simulink model "E5_Manual"  (R2019a)
settings: Solver=ode4  StartTime=0.0  StopTime=40  FixedStep=1e-3  RelTol=1e-2
libraries: simulink x2, simulink_extras x1
settings Model: Creator=anmay  LastModifiedBy=anmay
settings SolverCC: AlgebraicLoopSolver=LineSearch

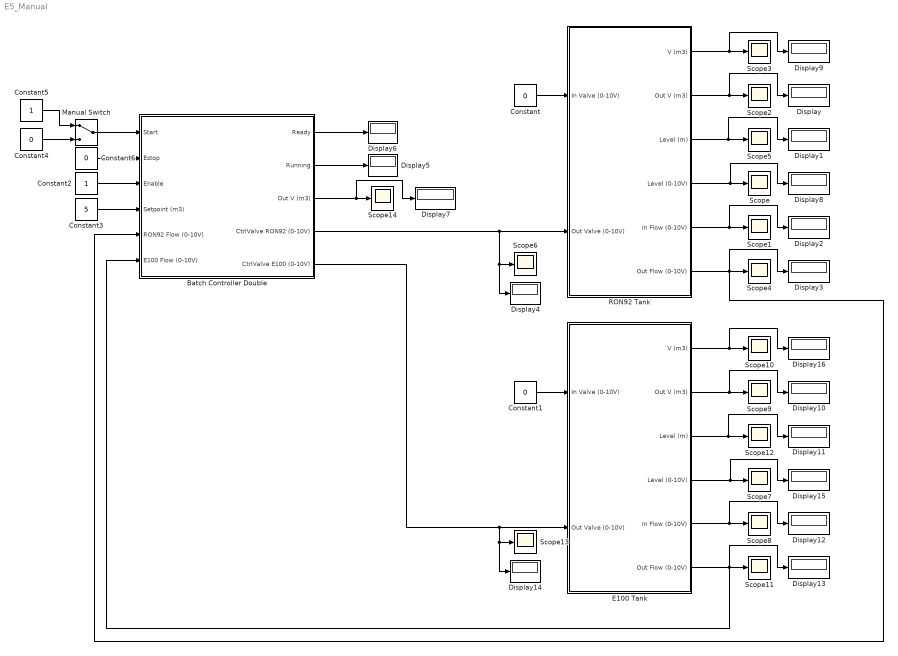
== system E5_Manual ==
  Batch Controller Double : Subsystem  mask{FlowMaxRON92=200, FlowMaxE100=100}
      mask prompts: FlowMaxRON92 "Lưu lượng tối đa RON92 (van mở 100%) (l/s)"; FlowMaxE100 "Lưu lượng tối đa E100 (van mở 100%) (l/s)"
  Constant{,1,4,6} (4 alike) : Constant  Value=0
  Constant2 : Constant
  Constant3 : Constant  Value=5
  Constant5 : Constant
  Display{,1..16} (17 alike) : Display
  E100 Tank : Subsystem  mask{InitialLevel=15, TankHeight=25, FlowMax=50, BaseArea=10, Tqt=0.1, EnableNoise=off, VarNoise=20}
      mask prompts: InitialLevel "Mức nhiên liệu ban đầu (m)"; TankHeight "Chiều cao của bể (m)"; FlowMax "Lưu lượng tối đa (van mở 100%) (l/s)"; BaseArea "Diện tích đáy (m2)"; Tqt "Hằng số quán tính của van (s)"; EnableNoise "Tạo nhiễu"; VarNoise "Phương sai của bộ tạo nhiễu"
  Manual Switch : ManualSwitch
  RON92 Tank : Subsystem  mask{InitialLevel=15, TankHeight=25, FlowMax=200, BaseArea=10, Tqt=0.2, EnableNoise=off, VarNoise=20}
      mask prompts: InitialLevel "Mức nhiên liệu ban đầu (m)"; TankHeight "Chiều cao của bể (m)"; FlowMax "Lưu lượng tối đa (van mở 100%) (l/s)"; BaseArea "Diện tích đáy (m2)"; Tqt "Hằng số quán tính của van (s)"; EnableNoise "Tạo nhiễu"; VarNoise "Phương sai của bộ tạo nhiễu"
  Scope{,1..14} (15 alike) : Scope
  wires:
  RON92 Tank/1(V (m3)) -> Display9/1, Scope3/1
  RON92 Tank/2(Out V (m3)) -> Scope2/1, Display/1
  RON92 Tank/3(Level (m)) -> Scope5/1, Display1/1
  RON92 Tank/6(Out Flow (0-10V)) -> Batch Controller Double/5(RON92 Flow (0-10V)), Display3/1, Scope4/1
  Batch Controller Double/4(CtrlValve RON92 (0-10V)) -> RON92 Tank/2(Out Valve (0-10V)), Display4/1, Scope6/1
  Batch Controller Double/2(Running) -> Display5/1
  RON92 Tank/4(Level (0-10V)) -> Scope/1, Display8/1
  Batch Controller Double/1(Ready) -> Display6/1
  RON92 Tank/5(In Flow (0-10V)) -> Display2/1, Scope1/1
  Constant/1 -> RON92 Tank/1(In Valve (0-10V))
  E100 Tank/5(In Flow (0-10V)) -> Display12/1, Scope8/1
  E100 Tank/3(Level (m)) -> Scope12/1, Display11/1
  E100 Tank/4(Level (0-10V)) -> Scope7/1, Display15/1
  Batch Controller Double/5(CtrlValve E100 (0-10V)) -> E100 Tank/2(Out Valve (0-10V)), Display14/1, Scope13/1
  E100 Tank/6(Out Flow (0-10V)) -> Batch Controller Double/6(E100 Flow (0-10V)), Display13/1, Scope11/1
  E100 Tank/1(V (m3)) -> Display16/1, Scope10/1
  Constant1/1 -> E100 Tank/1(In Valve (0-10V))
  E100 Tank/2(Out V (m3)) -> Scope9/1, Display10/1
  Constant4/1 -> Manual Switch/2
  Constant5/1 -> Manual Switch/1
  Constant2/1 -> Batch Controller Double/3(Enable)
  Constant6/1 -> Batch Controller Double/2(Estop)
  Constant3/1 -> Batch Controller Double/4(Setpoint (m3))
  Manual Switch/1 -> Batch Controller Double/1(Start)
  Batch Controller Double/3(Out V (m3)) -> Display7/1, Scope14/1

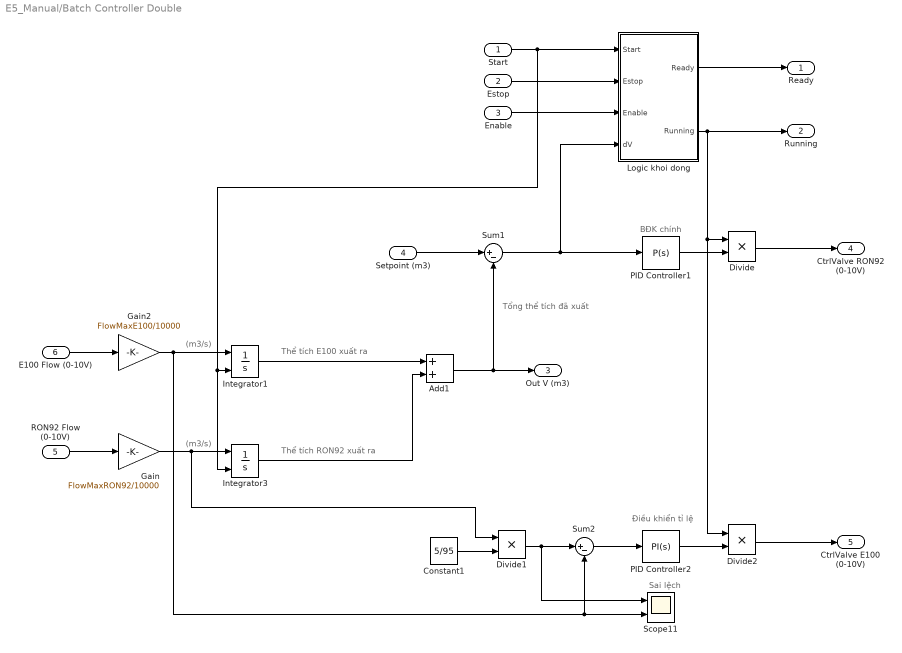
== system E5_Manual/Batch Controller Double ==
  note: (m3/s)
  note: BĐK chính
  note: Tổng thể tích đã xuất
  note: Điều khiển tỉ lệ
  note: Sai lệch
  note: Thể tích RON92 xuất ra
  note: Thể tích E100 xuất ra
  note: (m3/s)
  Start : Inport
  Estop : Inport  Port=2
  Enable : Inport  Port=3
  Setpoint (m3) : Inport  Port=4
  RON92 Flow (0-10V) : Inport  Port=5
  E100 Flow (0-10V) : Inport  Port=6
  Add1 : Sum
  Constant1 : Constant  Value=5/95
  Divide : Product  Inputs=**
  Divide1 : Product  Inputs=**
  Divide2 : Product  Inputs=**
  Gain : Gain  Gain=FlowMaxRON92/10000
  Gain2 : Gain  Gain=FlowMaxE100/10000
  Integrator1 : Integrator  ExternalReset=rising
  Integrator3 : Integrator  ExternalReset=rising
  Logic khoi dong : Subsystem
  PID Controller1 : simulink/Continuous/PID Controller  Controller=P  Form=Parallel  TimeDomain=Continuous-time  SampleTime=-1  IntegratorMethod=Forward Euler  FilterMethod=Forward Euler  ControllerParametersSource=internal  P=10  I=1  D=0  UseFilter=on  N=100  TunerSelectOption=Transfer Function Based (PID Tuner App)  InitialConditionSource=internal  InitialConditionForIntegrator=0  InitialConditionForFilter=0  DifferentiatorICPrevScaledInput=0  ExternalReset=none  TrackingMode=off  Kt=1  LimitOutput=on  UpperSaturationLimit=10  LowerSaturationLimit=0  LinearizeAsGain=on  AntiWindupMode=none  Kb=1  POutMin=[]  POutMax=[]  IOutMin=[]  IOutMax=[]  DOutMin=[]  DOutMax=[]  NOutMin=[]  NOutMax=[]  SumOutMin=[]  SumOutMax=[]  SaturationOutMin=[]  SaturationOutMax=[]  PParamMin=[]  PParamMax=[]  IParamMin=[]  IParamMax=[]  DParamMin=[]  DParamMax=[]  NParamMin=[]  NParamMax=[]  KbParamMin=[]  KbParamMax=[]  KtParamMin=[]  KtParamMax=[]  KbOutMin=[]  KbOutMax=[]  KtOutMin=[]  KtOutMax=[]  IntegratorOutMin=[]  IntegratorOutMax=[]  FilterOutMin=[]  FilterOutMax=[]  SumI1OutMin=[]  SumI1OutMax=[]  SumI2OutMin=[]  SumI2OutMax=[]  SumI3OutMin=[]  SumI3OutMax=[]  SumI4OutMin=[]  SumI4OutMax=[]  SumDOutMin=[]  SumDOutMax=[]  DifferentiatorOutMin=[]  DifferentiatorOutMax=[]  FilterDiffOutCoefMin=[]  FilterDiffOutCoefMax=[]  ReciprocalOutMin=[]  ReciprocalOutMax=[]  SumDenOutMin=[]  SumDenOutMax=[]  SumNumOutMin=[]  SumNumOutMax=[]  DivideOutMin=[]  DivideOutMax=[]  IntegratorContinuousStateAttributes=''  IntegratorStateMustResolveToSignalObject=off  IntegratorRTWStateStorageClass=Auto  FilterContinuousStateAttributes=''  FilterStateMustResolveToSignalObject=off  FilterRTWStateStorageClass=Auto  ParallelPVariant=InternalParameters  IdealPVariant=Disabled  IVariant=Disabled  DVariant=Disabled  IntegratorVariant=Disabled  SatVariant=Enabled  AWVariant=Disabled  PCopyVariant=Disabled  TRVariant=Disabled  FdbkBlocksVariant=Forward  IdealPFdbkVariant=Disabled  SatFdbkVariant=Disabled  DerivativeFilterVariant=Disabled  NVariant=Disabled  NCopyVariant=Disabled_SignalSpec  FilterICVariant=Disabled  IntegratorICVariant=Disabled  ExternalResetVariant=Disabled  TRSumVariant=Passthrough  SumFdbkVariant=Disabled  SumVariant=Passthrough_P
  PID Controller2 : simulink/Continuous/PID Controller  Controller=PI  Form=Parallel  TimeDomain=Continuous-time  SampleTime=-1  IntegratorMethod=Forward Euler  FilterMethod=Forward Euler  ControllerParametersSource=internal  P=200  I=1500  D=30  UseFilter=on  N=100  TunerSelectOption=Transfer Function Based (PID Tuner App)  InitialConditionSource=internal  InitialConditionForIntegrator=0  InitialConditionForFilter=0  DifferentiatorICPrevScaledInput=0  ExternalReset=none  TrackingMode=off  Kt=1  LimitOutput=on  UpperSaturationLimit=10  LowerSaturationLimit=0  LinearizeAsGain=on  AntiWindupMode=none  Kb=1  POutMin=[]  POutMax=[]  IOutMin=[]  IOutMax=[]  DOutMin=[]  DOutMax=[]  NOutMin=[]  NOutMax=[]  SumOutMin=[]  SumOutMax=[]  SaturationOutMin=[]  SaturationOutMax=[]  PParamMin=[]  PParamMax=[]  IParamMin=[]  IParamMax=[]  DParamMin=[]  DParamMax=[]  NParamMin=[]  NParamMax=[]  KbParamMin=[]  KbParamMax=[]  KtParamMin=[]  KtParamMax=[]  KbOutMin=[]  KbOutMax=[]  KtOutMin=[]  KtOutMax=[]  IntegratorOutMin=[]  IntegratorOutMax=[]  FilterOutMin=[]  FilterOutMax=[]  SumI1OutMin=[]  SumI1OutMax=[]  SumI2OutMin=[]  SumI2OutMax=[]  SumI3OutMin=[]  SumI3OutMax=[]  SumI4OutMin=[]  SumI4OutMax=[]  SumDOutMin=[]  SumDOutMax=[]  DifferentiatorOutMin=[]  DifferentiatorOutMax=[]  FilterDiffOutCoefMin=[]  FilterDiffOutCoefMax=[]  ReciprocalOutMin=[]  ReciprocalOutMax=[]  SumDenOutMin=[]  SumDenOutMax=[]  SumNumOutMin=[]  SumNumOutMax=[]  DivideOutMin=[]  DivideOutMax=[]  IntegratorContinuousStateAttributes=''  IntegratorStateMustResolveToSignalObject=off  IntegratorRTWStateStorageClass=Auto  FilterContinuousStateAttributes=''  FilterStateMustResolveToSignalObject=off  FilterRTWStateStorageClass=Auto  ParallelPVariant=InternalParameters  IdealPVariant=Disabled  IVariant=InternalParameters  DVariant=Disabled  IntegratorVariant=Continuous  SatVariant=Enabled  AWVariant=Passthrough  PCopyVariant=Disabled  TRVariant=Disabled  FdbkBlocksVariant=Forward  IdealPFdbkVariant=Disabled  SatFdbkVariant=Disabled  DerivativeFilterVariant=Disabled  NVariant=Disabled  NCopyVariant=Disabled_SignalSpec  FilterICVariant=Disabled  IntegratorICVariant=InternalICs  ExternalResetVariant=Disabled  TRSumVariant=Passthrough  SumFdbkVariant=Disabled  SumVariant=Sum_PI
  Scope11 : Scope  NumInputPorts=2
  Sum1 : Sum  Inputs=|+-
  Sum2 : Sum  Inputs=|+-
  Ready : Outport
  Running : Outport  Port=2
  Out V (m3) : Outport  Port=3
  CtrlValve RON92 (0-10V) : Outport  Port=4
  CtrlValve E100 (0-10V) : Outport  Port=5
  wires:
  RON92 Flow (0-10V)/1 -> Gain/1
  Logic khoi dong/2(Running) -> Running/1, Divide2/1, Divide/1
  Estop/1 -> Logic khoi dong/2(Estop)
  Start/1 -> Integrator1/2, Integrator3/2, Logic khoi dong/1(Start)
  Enable/1 -> Logic khoi dong/3(Enable)
  Logic khoi dong/1(Ready) -> Ready/1
  Constant1/1 -> Divide1/2
  Add1/1 -> Out V (m3)/1, Sum1/2
  Sum2/1 -> PID Controller2/1
  Sum1/1 -> Logic khoi dong/4(dV), PID Controller1/1
  Divide1/1 -> Scope11/1, Sum2/1
  Integrator3/1 -> Add1/2
  Gain/1 -> Divide1/1, Integrator3/1
  Gain2/1 -> Sum2/2, Scope11/2, Integrator1/1
  E100 Flow (0-10V)/1 -> Gain2/1
  Integrator1/1 -> Add1/1
  Setpoint (m3)/1 -> Sum1/1
  PID Controller1/1 -> Divide/2
  PID Controller2/1 -> Divide2/2
  Divide/1 -> CtrlValve RON92 (0-10V)/1
  Divide2/1 -> CtrlValve E100 (0-10V)/1

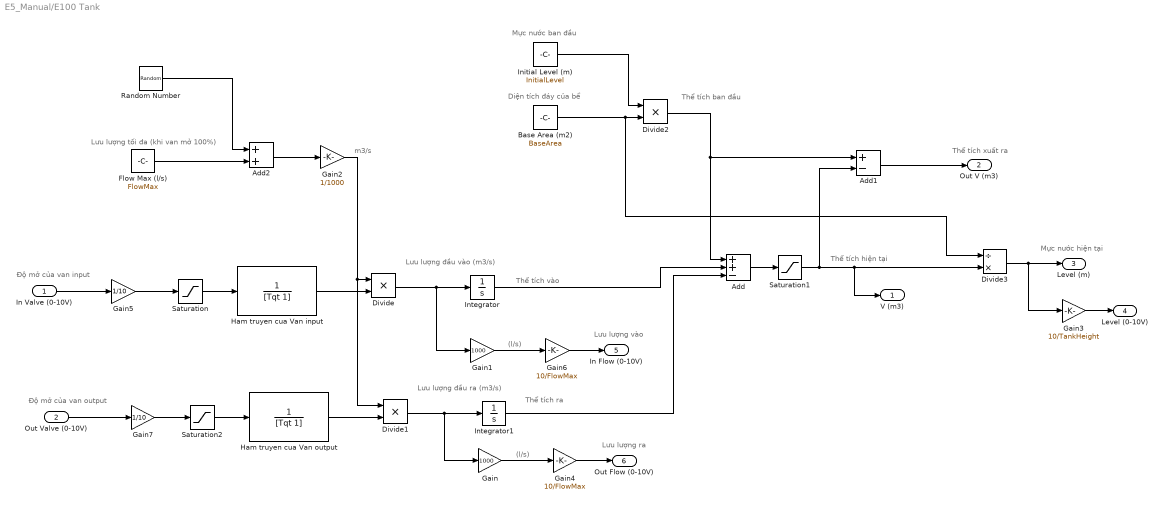
== system E5_Manual/E100 Tank ==
  note: (l/s)
  note: m3/s
  note: Lưu lượng ra
  note: Thể tích xuất ra
  note: Thể tích hiện tại
  note: Mực nước hiện tại
  note: Thể tích
      | ban đầu
  note: Mực nước ban đầu
  note: Diện tích đáy của bể
  note: Lưu lượng tối đa (khi van mở 100%)
  note: Độ mở của van output
  note: Thể tích ra
  note: Lưu lượng
      | đầu ra (m3/s)
  note: Thể tích vào
  note: Độ mở của van input
  note: Lưu lượng
      | đầu vào (m3/s)
  note: (l/s)
  note: Lưu lượng vào
  In Valve (0-10V) : Inport
  Out Valve (0-10V) : Inport  Port=2
  Add : Sum  Inputs=++-
  Add1 : Sum  Inputs=+-
  Add2 : Sum
  Base Area (m2) : Constant  Value=BaseArea
  Divide : Product  Inputs=**
  Divide1 : Product  Inputs=**
  Divide2 : Product  Inputs=**
  Divide3 : Product  Inputs=/*
  Flow Max (l/s) : Constant  Value=FlowMax
  Gain : Gain  Gain=1000
  Gain1 : Gain  Gain=1000
  Gain2 : Gain  Gain=1/1000
  Gain3 : Gain  Gain=10/TankHeight
  Gain4 : Gain  Gain=10/FlowMax
  Gain5 : Gain  Gain=1/10
  Gain6 : Gain  Gain=10/FlowMax
  Gain7 : Gain  Gain=1/10
  Ham truyen cua Van input : TransferFcn  Denominator=[Tqt 1]
  Ham truyen cua Van output : TransferFcn  Denominator=[Tqt 1]
  Initial Level (m) : Constant  Value=InitialLevel
  Integrator : Integrator
  Integrator1 : Integrator
  "Random Number " : RandomNumber  Variance=VarNoise*EnableNoise  SampleTime=0.5
  Saturation : Saturate  UpperLimit=1  LowerLimit=0
  Saturation1 : Saturate  UpperLimit=TankHeight*BaseArea  LowerLimit=0
  Saturation2 : Saturate  UpperLimit=1  LowerLimit=0
  V (m3) : Outport
  Out V (m3) : Outport  Port=2
  Level (m) : Outport  Port=3
  Level (0-10V) : Outport  Port=4
  In Flow (0-10V) : Outport  Port=5
  Out Flow (0-10V) : Outport  Port=6
  wires:
  Base Area (m2)/1 -> Divide3/1, Divide2/2
  Initial Level (m)/1 -> Divide2/1
  Divide3/1 -> Gain3/1, Level (m)/1
  Divide2/1 -> Add1/1, Add/1
  Add/1 -> Saturation1/1
  Saturation1/1 -> Add1/2, V (m3)/1, Divide3/2
  Add1/1 -> Out V (m3)/1
  Saturation2/1 -> Ham truyen cua Van output/1
  Ham truyen cua Van output/1 -> Divide1/2
  Divide1/1 -> Gain/1, Integrator1/1
  Gain3/1 -> Level (0-10V)/1
  Gain4/1 -> Out Flow (0-10V)/1
  Gain/1 -> Gain4/1
  Gain7/1 -> Saturation2/1
  Out Valve (0-10V)/1 -> Gain7/1
  "Random Number "/1 -> Add2/1
  Add2/1 -> Gain2/1
  Flow Max (l/s)/1 -> Add2/2
  Integrator/1 -> Add/2
  Gain2/1 -> Divide1/1, Divide/1
  Ham truyen cua Van input/1 -> Divide/2
  Saturation/1 -> Ham truyen cua Van input/1
  Gain5/1 -> Saturation/1
  In Valve (0-10V)/1 -> Gain5/1
  Integrator1/1 -> Add/3
  Divide/1 -> Gain1/1, Integrator/1
  Gain6/1 -> In Flow (0-10V)/1
  Gain1/1 -> Gain6/1

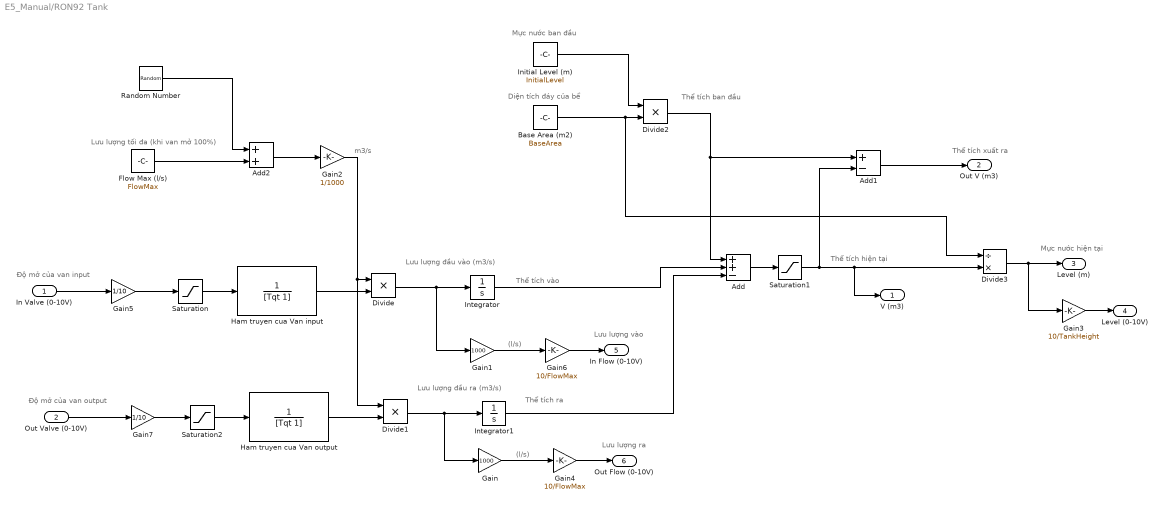
== system E5_Manual/RON92 Tank ==
  note: (l/s)
  note: m3/s
  note: Lưu lượng ra
  note: Thể tích xuất ra
  note: Thể tích hiện tại
  note: Mực nước hiện tại
  note: Thể tích
      | ban đầu
  note: Mực nước ban đầu
  note: Diện tích đáy của bể
  note: Lưu lượng tối đa (khi van mở 100%)
  note: Độ mở của van output
  note: Thể tích ra
  note: Lưu lượng
      | đầu ra (m3/s)
  note: Thể tích vào
  note: Độ mở của van input
  note: Lưu lượng
      | đầu vào (m3/s)
  note: (l/s)
  note: Lưu lượng vào
  In Valve (0-10V) : Inport
  Out Valve (0-10V) : Inport  Port=2
  Add : Sum  Inputs=++-
  Add1 : Sum  Inputs=+-
  Add2 : Sum
  Base Area (m2) : Constant  Value=BaseArea
  Divide : Product  Inputs=**
  Divide1 : Product  Inputs=**
  Divide2 : Product  Inputs=**
  Divide3 : Product  Inputs=/*
  Flow Max (l/s) : Constant  Value=FlowMax
  Gain : Gain  Gain=1000
  Gain1 : Gain  Gain=1000
  Gain2 : Gain  Gain=1/1000
  Gain3 : Gain  Gain=10/TankHeight
  Gain4 : Gain  Gain=10/FlowMax
  Gain5 : Gain  Gain=1/10
  Gain6 : Gain  Gain=10/FlowMax
  Gain7 : Gain  Gain=1/10
  Ham truyen cua Van input : TransferFcn  Denominator=[Tqt 1]
  Ham truyen cua Van output : TransferFcn  Denominator=[Tqt 1]
  Initial Level (m) : Constant  Value=InitialLevel
  Integrator : Integrator
  Integrator1 : Integrator
  "Random Number " : RandomNumber  Variance=VarNoise*EnableNoise  SampleTime=0.5
  Saturation : Saturate  UpperLimit=1  LowerLimit=0
  Saturation1 : Saturate  UpperLimit=TankHeight*BaseArea  LowerLimit=0
  Saturation2 : Saturate  UpperLimit=1  LowerLimit=0
  V (m3) : Outport
  Out V (m3) : Outport  Port=2
  Level (m) : Outport  Port=3
  Level (0-10V) : Outport  Port=4
  In Flow (0-10V) : Outport  Port=5
  Out Flow (0-10V) : Outport  Port=6
  wires:
  Base Area (m2)/1 -> Divide3/1, Divide2/2
  Initial Level (m)/1 -> Divide2/1
  Divide3/1 -> Gain3/1, Level (m)/1
  Divide2/1 -> Add1/1, Add/1
  Add/1 -> Saturation1/1
  Saturation1/1 -> Add1/2, V (m3)/1, Divide3/2
  Add1/1 -> Out V (m3)/1
  Saturation2/1 -> Ham truyen cua Van output/1
  Ham truyen cua Van output/1 -> Divide1/2
  Divide1/1 -> Gain/1, Integrator1/1
  Gain3/1 -> Level (0-10V)/1
  Gain4/1 -> Out Flow (0-10V)/1
  Gain/1 -> Gain4/1
  Gain7/1 -> Saturation2/1
  Out Valve (0-10V)/1 -> Gain7/1
  "Random Number "/1 -> Add2/1
  Add2/1 -> Gain2/1
  Flow Max (l/s)/1 -> Add2/2
  Integrator/1 -> Add/2
  Gain2/1 -> Divide1/1, Divide/1
  Ham truyen cua Van input/1 -> Divide/2
  Saturation/1 -> Ham truyen cua Van input/1
  Gain5/1 -> Saturation/1
  In Valve (0-10V)/1 -> Gain5/1
  Integrator1/1 -> Add/3
  Divide/1 -> Gain1/1, Integrator/1
  Gain6/1 -> In Flow (0-10V)/1
  Gain1/1 -> Gain6/1

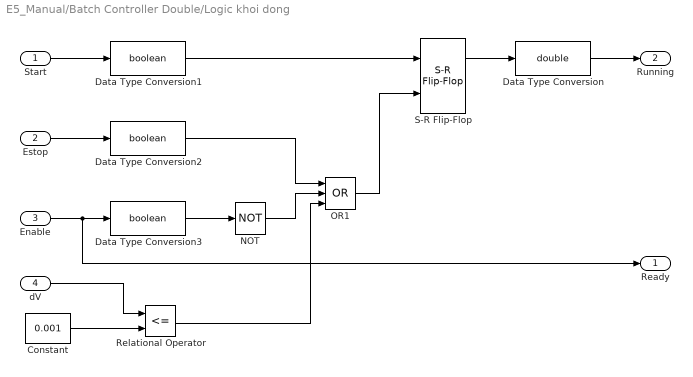
== system E5_Manual/Batch Controller Double/Logic khoi dong ==
  Start : Inport
  Estop : Inport  Port=2
  Enable : Inport  Port=3
  dV : Inport  Port=4
  Constant : Constant  Value=0.001
  Data Type Conversion : DataTypeConversion  OutDataTypeStr=double
  Data Type Conversion1 : DataTypeConversion  OutDataTypeStr=boolean
  Data Type Conversion2 : DataTypeConversion  OutDataTypeStr=boolean
  Data Type Conversion3 : DataTypeConversion  OutDataTypeStr=boolean
  NOT : Logic  Operator=NOT  IconShape=distinctive  AllPortsSameDT=off  OutDataTypeStr=boolean
  OR1 : Logic  Operator=OR  Inputs=3  IconShape=distinctive  AllPortsSameDT=off  OutDataTypeStr=boolean
  Relational Operator : RelationalOperator  Operator=<=  OutDataTypeStr=boolean  RndMeth=Simplest
  S-R Flip-Flop : simulink_extras/Flip Flops/S-R Flip-Flop  initial_condition=0
  Ready : Outport
  Running : Outport  Port=2
  wires:
  Constant/1 -> Relational Operator/2
  dV/1 -> Relational Operator/1
  Start/1 -> Data Type Conversion1/1
  Estop/1 -> Data Type Conversion2/1
  Data Type Conversion2/1 -> OR1/1
  Data Type Conversion1/1 -> S-R Flip-Flop/1
  OR1/1 -> S-R Flip-Flop/2
  Data Type Conversion3/1 -> NOT/1
  NOT/1 -> OR1/2
  Relational Operator/1 -> OR1/3
  S-R Flip-Flop/1 -> Data Type Conversion/1
  Data Type Conversion/1 -> Running/1
  Enable/1 -> Ready/1, Data Type Conversion3/1
